simulink model "Kinematic_geometric_control"  (R2025b)
settings: Solver=VariableStepAuto  StartTime=0.0  StopTime=5  RelTol=1e-3
settings Model: Creator=lucag  LastModifiedBy=lucag

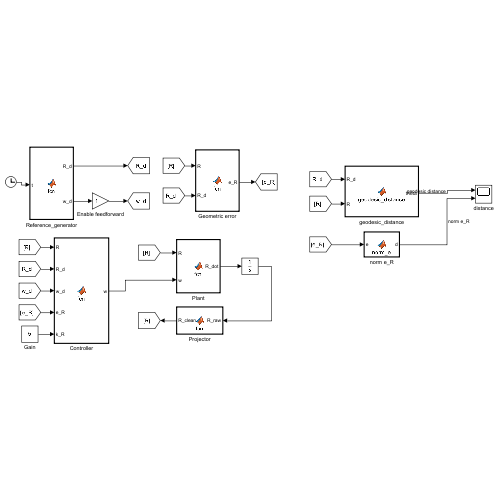
[thumbnail: Simulink's stored preview of the top-level diagram]
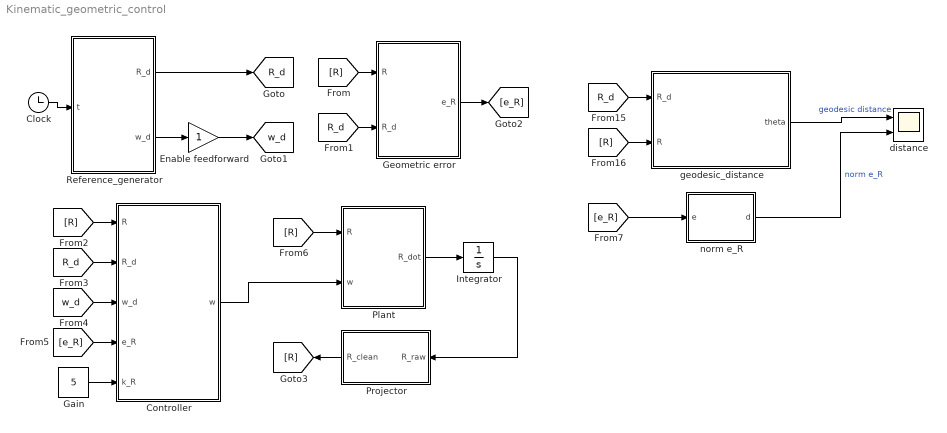
== system Kinematic_geometric_control ==
  Clock : Clock
  Controller : MATLAB Function  TreatAsAtomicUnit=on
  Enable feedforward : Gain
  Gain : Constant  Value=5
  Geometric error : MATLAB Function  TreatAsAtomicUnit=on
  Integrator : Integrator  InitialCondition=eye(3)
  Plant : MATLAB Function  TreatAsAtomicUnit=on
  Projector : MATLAB Function  TreatAsAtomicUnit=on
  Reference_generator : MATLAB Function  TreatAsAtomicUnit=on
  distance : Scope  NumInputPorts=2
      settings: ActiveDisplayYMinimum=-22.47727985999714  ActiveDisplayYMaximum=202.29747554000065
  geodesic_distance : MATLAB Function  TreatAsAtomicUnit=on
  norm e_R : MATLAB Function  TreatAsAtomicUnit=on
  tag scope: R_d=global, w_d=global
  wires:
  Plant/1(R_dot) -> Integrator/1
  Controller/1(w) -> Plant/2(w)
  Gain/1 -> Controller/5(k_R)
  Integrator/1 -> Projector/1(R_raw)
  [R] -> Geometric error/1(R)
  [R_d] -> Geometric error/2(R_d)
  Geometric error/1(e_R) -> [e_R]
  [R] -> Controller/1(R)
  [R_d] -> Controller/2(R_d)
  [w_d] -> Controller/3(w_d)
  [e_R] -> Controller/4(e_R)
  [R] -> Plant/1(R)
  Projector/1(R_clean) -> [R]
  Enable feedforward/1 -> [w_d]
  Clock/1 -> Reference_generator/1(t)
  Reference_generator/2(w_d) -> Enable feedforward/1
  Reference_generator/1(R_d) -> [R_d]
  [e_R] -> norm e_R/1(e)
  norm e_R/1(d) -> distance/2  "norm e_R"
  [R] -> geodesic_distance/2(R)
  [R_d] -> geodesic_distance/1(R_d)
  geodesic_distance/1(theta) -> distance/1  "geodesic distance"

== matlab function Kinematic_geometric_control/Controller ==
  data: R input; w output; R_d input; w_d input; e_R input; k_R input
function w = fcn(R, R_d, w_d, e_R, k_R)

    % Feedforward term
    feedforward = R' * R_d * w_d;

    % Proportional feedback term
    feedback = -k_R * e_R;

    % Total control effort
    w = feedforward + feedback;
end

== matlab function Kinematic_geometric_control/Geometric error ==
  data: R input; e_R output; R_d input
function e_R = fcn(R, R_d)
    
    % Calculate the skew-symmetric error matrix
    S = 0.5 * (R_d' * R - R' * R_d);

    % Apply the vee map to extract the vector
    e_R = [S(3,2); S(1,3); S(2,1)];
    
end

== matlab function Kinematic_geometric_control/Plant ==
  data: R input; R_dot output; w input
function R_dot = fcn(R, w)
    % Apply the hat map to omega
    omega_hat = [   0,      -w(3),  w(2);
                 w(3),      0,     -w(1);
                -w(2),  w(1),      0    ];

    % Bilinear differential equation
    R_dot = R * omega_hat;
end

== matlab function Kinematic_geometric_control/Reference_generator ==
  data: R_d output; w_d output; t input
function [R_d, w_d] = fcn(t)
% % Time varying angles Roll (phi), Pitch (theta) and Yaw (psi) that
% % generates a time varying reference matrix R_d(t)
% phi = pi/4*sin(t);
% theta = pi/4*sin(t);
% psi = pi/4*sin(t);
% 
% % These derivatives are used to compute R_d_dot
% phi_dot = pi/4*cos(t);
% theta_dot = pi/4*cos(t);
% psi_dot = pi/4*cos(t);
% 
% angles_d = [phi, theta, psi]';
% 
% R11 = cos(psi)*cos(theta);
% R12 = cos(psi)*sin(theta)*sin(phi) - sin(psi)*cos(phi);
% R13 = cos(psi)*sin(theta)*cos(phi) + sin(psi)*sin(phi);
% R21 = sin(psi)*cos(theta);
% R22 = sin(psi)*sin(theta)*sin(phi) + cos(psi)*cos(phi);
% R23 = sin(psi)*sin(theta)*cos(phi) - cos(psi)*sin(phi);
% R31 = -sin(theta);
% R32 = cos(theta)*sin(phi);
% R33 = cos(theta)*cos(phi);
% 
% R_d = [R11 R12 R13;
%     R21 R22 R23;
%     R31 R32 R33];
% 
% % Compute the skew simmetric matrix of omega_d
% omega_d_hat = R_d'*compute_Rdot(phi, theta, psi, phi_dot, theta_dot, psi_dot);
% 
% % Extract the vector
% w_d = [omega_d_hat(3,2);
%     omega_d_hat(1,3);
%     omega_d_hat(2,1)];
% end
% 
% 
% function R_d_dot = compute_Rdot(phi, theta, psi, phi_dot, theta_dot, psi_dot)
% % The entry [R_d_dot]_ij is the time derivative of [R_d]_ij
% R11_dot = -psi_dot * sin(psi) * cos(theta) ...
%     - theta_dot * cos(psi) * sin(theta);
% 
% R12_dot =  phi_dot * (cos(psi) * sin(theta) * cos(phi) + sin(psi) * sin(phi)) ...
%     + theta_dot * (cos(psi) * cos(theta) * sin(phi)) ...
%     - psi_dot * (sin(psi) * sin(theta) * sin(phi) + cos(psi) * cos(phi));
% 
% R13_dot =  phi_dot * (-cos(psi) * sin(theta) * sin(phi) + sin(psi) * cos(phi)) ...
%     + theta_dot * (cos(psi) * cos(theta) * cos(phi)) ...
%     - psi_dot * (sin(psi) * sin(theta) * cos(phi) - cos(psi) * sin(phi));
% 
% R21_dot =  psi_dot * cos(psi) * cos(theta) ...
%     - theta_dot * sin(psi) * sin(theta);
% 
% R22_dot =  phi_dot * (sin(psi) * sin(theta) * cos(phi) - cos(psi) * sin(phi)) ...
%     + theta_dot * (sin(psi) * cos(theta) * sin(phi)) ...
%     + psi_dot * (cos(psi) * sin(theta) * sin(phi) - sin(psi) * cos(phi));
% 
% R23_dot =  phi_dot * (-sin(psi) * sin(theta) * sin(phi) - cos(psi) * cos(phi)) ...
%     + theta_dot * (sin(psi) * cos(theta) * cos(phi)) ...
%     + psi_dot * (cos(psi) * sin(theta) * cos(phi) + sin(psi) * sin(phi));
% 
% R31_dot = -theta_dot * cos(theta);
% 
% R32_dot =  phi_dot * cos(theta) * cos(phi) ...
%     - theta_dot * sin(theta) * sin(phi);
% 
% R33_dot = -phi_dot * cos(theta) * sin(phi) ...
%     - theta_dot * sin(theta) * cos(phi);
% 
% % --- Assemble Matrix ---
% R_d_dot = [R11_dot, R12_dot, R13_dot;
%     R21_dot, R22_dot, R23_dot;
%     R31_dot, R32_dot, R33_dot];

% Implementation of paper time-dependent reference
phi = 0.999*pi + 0.5*t;
theta = 0.1*t^2;
psi = -0.2*t + 0.5*t^2;

phi_dot = 0.5;
theta_dot = 2*0.1*t;
psi_dot = t-0.2;

phi_ddot = 0;
theta_ddot = 0.2;
psi_ddot = 1;

angles_d = [phi, theta, psi]';

R11 = cos(psi)*cos(theta);
R12 = cos(psi)*sin(theta)*sin(phi) - sin(psi)*cos(phi);
R13 = cos(psi)*sin(theta)*cos(phi) + sin(psi)*sin(phi);
R21 = sin(psi)*cos(theta);
R22 = sin(psi)*sin(theta)*sin(phi) + cos(psi)*cos(phi);
R23 = sin(psi)*sin(theta)*cos(phi) - cos(psi)*sin(phi);
R31 = -sin(theta);
R32 = cos(theta)*sin(phi);
R33 = cos(theta)*cos(phi);

R_d = [R11 R12 R13;
    R21 R22 R23;
    R31 R32 R33];

% 4. Compute Desired Angular Velocity (omega_d)
omega_d_1 = phi_dot - psi_dot*sin(theta);
omega_d_2 = theta_dot*cos(phi) + psi_dot*sin(phi)*cos(theta);
omega_d_3 = -theta_dot*sin(phi) + psi_dot*cos(phi)*cos(theta);

w_d = [omega_d_1, omega_d_2, omega_d_3]';
end

== matlab function Kinematic_geometric_control/Projector ==
  data: R_raw input; R_clean output
function R_clean = fcn(R_raw)
    % This script is used to project back on SO(3) the output of the
    % integrator, which can no longer be a valid rotation matrix due to
    % numerical intgration errors.

    % Perform SVD
    [U, ~, V] = svd(R_raw);
    
    % Reconstruct the closest orthogonal matrix
    R_clean = U * V';
    
    % Ensure determinant is +1 (proper rotation, not reflection)
    if det(R_clean) < 0
        U(:,3) = -U(:,3);
        R_clean = U * V';
    end
end

== matlab function Kinematic_geometric_control/geodesic_distance ==
  data: theta output; R_d input; R input
% GEODESIC_DISTANCE Calculates the shortest angle between two orientations

% Computes the relative rotation matrix (R_d' * R) and extracts the
% single rotation angle using the matrix trace property. This avoids
% the wrapping and singularity issues of Euler angles.

function theta = geodesic_distance(R_d, R)

R = R_d' * R;
theta = acos((trace(R) - 1)/2);
theta = rad2deg(theta);

end

== matlab function Kinematic_geometric_control/norm e_R ==
  data: d output; e input
function d = norm_e(e)

d = norm(e);

end
